simulink model "gazebo_controller"  (R2022a)
settings: Solver=FixedStepAuto  StartTime=0.0  StopTime=10.0  RelTol=1e-3
model workspace (MAT data in the model file):
  SL_ROS_VariableLengthArrays_MaxSizes.CommonInfo.ArrayTruncateAction = 'EmitWarning'
  SL_ROS_VariableLengthArrays_MaxSizes.MsgTypeMap = containers.Map
  SL_ROS_VariableLengthArrays_MaxSizes.MsgTypeMap.serialization.keys = {'std_msgs/Float64MultiArray'}
  SL_ROS_VariableLengthArrays_MaxSizes.MsgTypeMap.serialization.values{1}.PropertyName = 'data'
  SL_ROS_VariableLengthArrays_MaxSizes.MsgTypeMap.serialization.values{1}.DataType = 'double'
  SL_ROS_VariableLengthArrays_MaxSizes.MsgTypeMap.serialization.values{1}.MaxLength = 6
  SL_ROS_VariableLengthArrays_MaxSizes.MsgTypeMap.serialization.uniformity = 0
  SL_ROS_VariableLengthArrays_MaxSizes.MsgTypeMap.serialization.keyType = 'char'
  SL_ROS_VariableLengthArrays_MaxSizes.MsgTypeMap.serialization.valueType = 'any'
values from neighbouring files (symbols this model uses):
  A = [0 1 0 0 0 0 0 0 0 0 0 0 0 0 0 0 0 0 ... (first row only)    [Effort_controller.m]
  Ad = discrete_plant.A    [Effort_controller.m]
  B = [ ... (first row only)    [Effort_controller.m]
  Bd = discrete_plant.B    [Effort_controller.m]
  C = [1 0 0 0 0 0 0 0 0 0 0 0 0 0 0 0 0 0 ... (first row only)    [Effort_controller.m]
  Cd = discrete_plant.C    [Effort_controller.m]
  L = place(Ad', Cd', poles_d)'    [Effort_controller.m]    (also in Lagrange_Model.m = vpa(L, 6); for2021a.m = (m5*((l2*cos(th1)*cos(th2)*th1d - l2*sin(th1)*sin(th2)*th2d )
libraries: ros2lib x3, robotgazebolib x2, simulink x1
settings Model: Creator=legacy  LastModifiedBy=legacy
settings OptimizationCC: EnhancedBackFolding=on  PassReuseOutputArgsAs=Individual arguments  ZeroExternalMemoryAtStartup=off  ZeroInternalMemoryAtStartup=off  MaxStackSize=64  OptimizeBlockOrder=speed  DifferentSizesBufferReuse=on  OptimizationCustomize=off  EfficientTunableParamExpr=on
settings DebuggingCC: ParameterTunabilityLossMsg=error
settings HardwareCC: ProdBitPerLong=64  ProdHWDeviceType=Intel->x86-64 (Linux 64)  UseEmbeddedCoderFeatures=off
settings SFSimCC: MATLABDynamicMemAlloc=off
settings RTWCC: SystemTargetFile=ert.tlc  HardwareBoard=Robot Operating System 2 (ROS 2)  TLCOptions="-aInlineSetEventsForThisBaseRateFcn=TLC_FALSE -aSuppressMultiTaskScheduler=TLC_FALSE  -aRateBasedStepFcn=0"  TemplateMakefile=ert_default_tmf  Toolchain=Colcon Tools  TargetLang=C++
settings CodeAppCC: ForceParamTrailComments=on  IgnoreCustomStorageClasses=off  OperatorAnnotations=on  SimulinkDataObjDesc=on  SFDataObjDesc=on  InsertBlockDesc=on
settings ERTTargetCC: CodeInterfacePackaging=C++ class  SupportNonInlinedSFcns=on  RootIOFormat=Structure reference

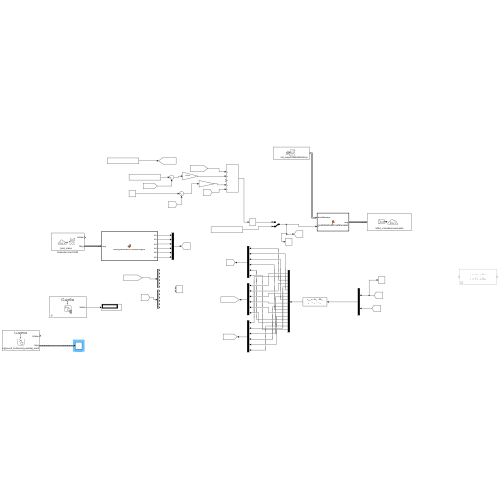
[thumbnail: Simulink's stored preview of the top-level diagram]
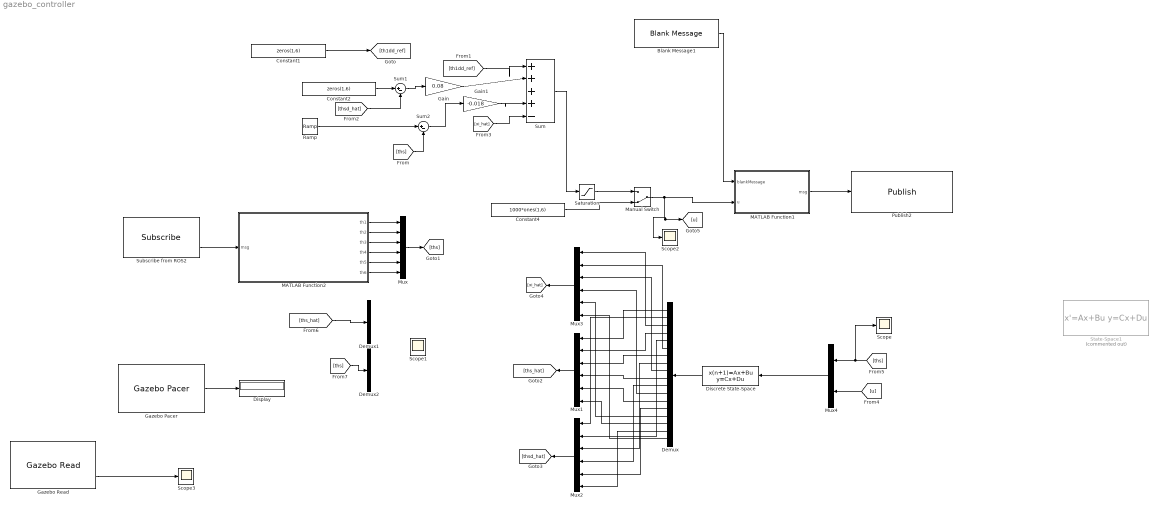
== system gazebo_controller ==
  Blank Message1 : ros2lib/Blank Message  messageClass=Message  entityType=std_msgs/Float64MultiArray  messageType=std_msgs/Float64MultiArray  SampleTime=0.01
      settings: SourceProductBaseCode=RR
  Constant1 : Constant  Value=zeros(1,6)
  Constant2 : Constant  Value=zeros(1,6)  SampleTime=0.01
  Constant4 : Constant  Value=1000*ones(1,6)  SampleTime=0.01
  Demux : Demux  Outputs=18
  Demux1 : Demux  Outputs=6
  Demux2 : Demux  Outputs=6
  Discrete State-Space : DiscreteStateSpace  A=Ad-L*Cd  B=[Bd L]  C=eye(18)  D=zeros(18,12)  SampleTime=0.01
  Display : Display
  Gain : Gain  Gain=0.08
  Gain1 : Gain  Gain=-0.018
  Gazebo Pacer : robotgazebolib/Gazebo Pacer  ResetBehavior=Reset Gazebo simulation time and scene  SampleTime=0.01
      settings: SourceProductBaseCode=RO
  Gazebo Read : robotgazebolib/Gazebo Read  topicSource=From Gazebo  topic=/gazebo/ground_truth/world_pose/big_arm/link_1  messageType=gazebo_msgs/Pose  sampleTime=0.01
      settings: SourceProductBaseCode=RO
  MATLAB Function1 : MATLAB Function  TreatAsAtomicUnit=on  SystemSampleTime=0.01
  MATLAB Function2 : MATLAB Function  TreatAsAtomicUnit=on  SystemSampleTime=0.01
  Manual Switch : ManualSwitch  CurrentSetting=0
  Mux{,1..3} (4 alike) : Mux  Inputs=6
  Mux4 : Mux  Inputs=2
  Publish2 : ros2lib/Publish  topicSource=Select from ROS network  topic=/effort_controllers/commands  messageType=std_msgs/Float64MultiArray  QOSHistory=Keep last  QOSDepth=1  QOSReliability=Reliable  QOSDurability=Volatile
      settings: SourceProductBaseCode=RR
  Ramp : simulink/Sources/Ramp  slope=[0.1, 0.1, 0.1, 0.1, 0.1, 0.1]  start=[1, 1, 1, 1, 1, 1]  InitialOutput=0
  Saturation : Saturate  UpperLimit=400*ones(1, 6)  LowerLimit=400*ones(1, 6)
  Scope : Scope
  Scope1 : Scope  NumInputPorts=2
  Scope2 : Scope
  Scope3 : Scope
  State-Space1 : StateSpace  Commented=on  A=A-L*C  B=[B L]  C=eye(18)  D=zeros(18, 12)  InitialCondition=0
  Subscribe from ROS2 : ros2lib/Subscribe  topicSource=Select from ROS network  topic=/joint_states  messageType=sensor_msgs/JointState  sampleTime=0.01  QOSHistory=Keep last  QOSDepth=1  QOSReliability=Reliable  QOSDurability=Volatile
      settings: SourceProductBaseCode=RR
  Sum : Sum  Inputs=|++++-
  Sum1 : Sum  Inputs=|+-
  Sum2 : Sum  Inputs=|+-
  wires:
  Demux/18 -> Mux3/6
  Demux/12 -> Mux3/4
  Demux/2 -> Mux2/1
  Blank Message1/1 -> MATLAB Function1/1(blankMessage)
  [u] -> Mux4/2
  [ths] -> Scope/1, Mux4/1
  [ths_hat] -> Demux1/1
  Sum/1 -> Saturation/1
  Gain1/1 -> Sum/4
  Demux/11 -> Mux2/4
  Mux4/1 -> Discrete State-Space/1
  Demux/3 -> Mux3/1
  Ramp/1 -> Sum2/1
  Sum1/1 -> Gain/1
  Saturation/1 -> Manual Switch/1
  Manual Switch/1 -> Scope2/1, [u], MATLAB Function1/2(u)
  MATLAB Function2/5(th5) -> Mux/5
  Demux/4 -> Mux1/2
  Mux/1 -> [ths]
  Sum2/1 -> Gain1/1
  [thsd_hat] -> Sum1/2
  Gazebo Pacer/1 -> Display/1
  Demux/7 -> Mux1/3
  Demux/1 -> Mux1/1
  MATLAB Function2/4(th4) -> Mux/4
  MATLAB Function2/2(th2) -> Mux/2
  Subscribe from ROS2/2 -> MATLAB Function2/1(msg)
  MATLAB Function1/1(msg) -> Publish2/1
  Mux2/1 -> [thsd_hat]
  Demux/16 -> Mux1/6
  Discrete State-Space/1 -> Demux/1
  Demux/17 -> Mux2/6
  Demux/13 -> Mux1/5
  Demux/14 -> Mux2/5
  [xi_hat] -> Sum/5
  Demux/8 -> Mux2/3
  Demux/15 -> Mux3/5
  Demux/10 -> Mux1/4
  Mux3/1 -> [xi_hat]
  MATLAB Function2/6(th6) -> Mux/6
  Constant1/1 -> [th1dd_ref]
  Gain/1 -> Sum/2
  Constant2/1 -> Sum1/1
  [th1dd_ref] -> Sum/1
  Mux1/1 -> [ths_hat]
  MATLAB Function2/3(th3) -> Mux/3
  Demux/9 -> Mux3/3
  Demux/5 -> Mux2/2
  [ths] -> Sum2/2
  MATLAB Function2/1(th1) -> Mux/1
  [ths] -> Demux2/1
  Demux/6 -> Mux3/2
  Constant4/1 -> Manual Switch/2
  Gazebo Read/2 -> Scope3/1

== matlab function gazebo_controller/MATLAB Function1 ==
  data: blankMessage input Bus: SL_Bus_std_msgs_Float64MultiArray; u input; msg output Bus: SL_Bus_std_msgs_Float64MultiArray
function msg = assignNestedArrayMessages(blankMessage,u)
%#codegen

msg = blankMessage;
msg.data = u;

msg.data_SL_Info.CurrentLength = uint32(6);

== matlab function gazebo_controller/MATLAB Function2 ==
  data: msg input Bus: SL_Bus_sensor_msgs_JointState; th1 output double; th2 output; th3 output; th4 output; th5 output; th6 output
function [th1, th2, th3, th4, th5, th6] = assignNestedArrayMessages(msg)
%#codegen
th1 = msg.position(6);
th2 = msg.position(1);
th3 = msg.position(2);
th4 = msg.position(3);
th5 = msg.position(4);
th6 = msg.position(5);
